simulink model "fw_sim"  (R2020a)
settings: Solver=ode4  StartTime=0.0  StopTime=45  FixedStep=0.01  RelTol=1e-3  EnableMultiTasking=on
undefined symbols (not defined in the file): ic_ned, ic_pqr, ic_rpy, ic_u, ic_uvw, wind
settings Model: Creator=fmina  LastModifiedBy=Chenhao
settings DataIOCC: SaveFormat=StructureWithTime  ReturnWorkspaceOutputs=off
settings OptimizationCC: LifeSpan=inf
settings DebuggingCC: SFUnexpectedBacktrackingDiag=warning  SFNoUnconditionalDefaultTransitionDiag=warning  SFExecutionAtInitializationDiag=none  ArithmeticOperatorsInVariantConditions=warning
settings HardwareCC: ProdBitPerSizeT=32  ProdBitPerPtrDiffT=32  ProdWordSize=32  ProdHWDeviceType=Specified
settings SFSimCC: SimUseLocalCustomCode=off  CustomCodeUndefinedFunction=UseInterfaceOnly
settings RTWCC: RTWUseLocalCustomCode=off
settings CodeAppCC: StateflowObjectComments=on
settings GRTTargetCC: TargetLangStandard=C89/C90 (ANSI)
settings ConfigComp: CovMetricSettings=dw  CovHtmlReporting=on  CovSaveCumulativeToWorkspaceVar=on  CovSaveSingleToWorkspaceVar=on  CovExternalEMLEnable=off

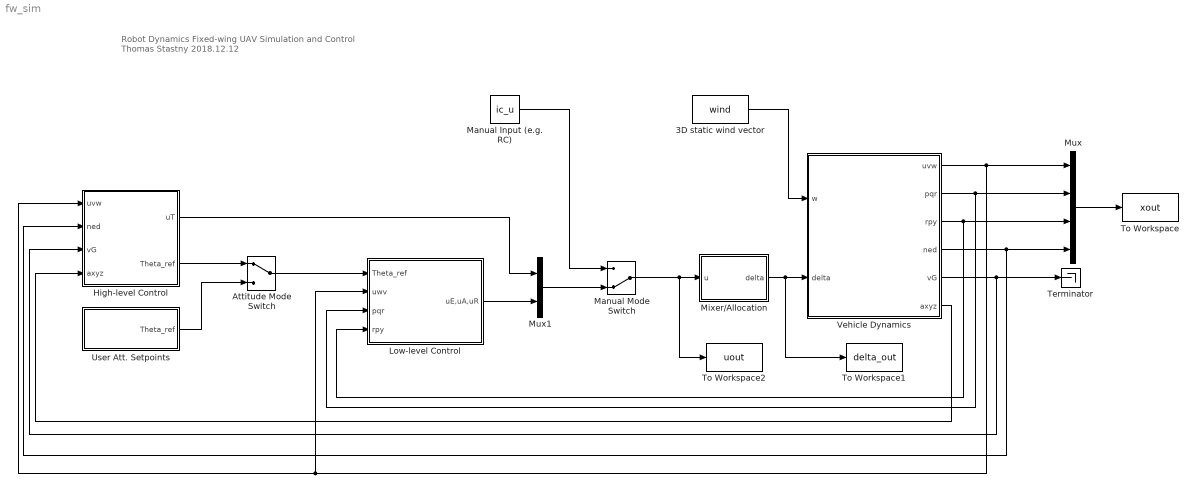
== system fw_sim ==
  note: Robot Dynamics
      | Fixed-wing UAV Simulation and Control
      |
      | Thomas Stastny
      | 2018.12.12
  3D static wind vector : Constant  Value=wind
  Attitude Mode Switch : ManualSwitch
  High-level Control : Subsystem
  Low-level Control : Subsystem
  Manual Input (e.g. RC) : Constant  Value=ic_u
  Manual Mode Switch : ManualSwitch  CurrentSetting=0
  Mixer/Allocation : MATLAB Function  TreatAsAtomicUnit=on
  Mux : Mux
  Mux1 : Mux  Inputs=2
  Terminator : Terminator
  To Workspace : ToWorkspace  VariableName=xout  SaveFormat=Structure With Time  SampleTime=-1
  To Workspace1 : ToWorkspace  VariableName=delta_out  SaveFormat=Structure With Time  SampleTime=-1
  To Workspace2 : ToWorkspace  VariableName=uout  SaveFormat=Structure With Time  SampleTime=-1
  User Att. Setpoints : Subsystem
  Vehicle Dynamics : Subsystem
  wires:
  3D static wind vector/1 -> Vehicle Dynamics/1(w)
  Mixer/Allocation/1(delta) -> To Workspace1/1, Vehicle Dynamics/2(delta)
  Mux/1 -> To Workspace/1
  Vehicle Dynamics/4(ned) -> High-level Control/2(ned), Mux/4
  Vehicle Dynamics/3(rpy) -> Low-level Control/4(rpy), Mux/3
  Vehicle Dynamics/1(uvw) -> Mux/1, Low-level Control/2(uwv), High-level Control/1(uvw)
  Vehicle Dynamics/2(pqr) -> Low-level Control/3(pqr), Mux/2
  Vehicle Dynamics/5(vG) -> High-level Control/3(vG), Terminator/1
  High-level Control/1(uT) -> Mux1/1
  Low-level Control/1(uE,uA,uR) -> Mux1/2
  Manual Mode Switch/1 -> To Workspace2/1, Mixer/Allocation/1(u)
  Manual Input (e.g. RC)/1 -> Manual Mode Switch/1
  Mux1/1 -> Manual Mode Switch/2
  Vehicle Dynamics/6(axyz) -> High-level Control/4(axyz)
  Attitude Mode Switch/1 -> Low-level Control/1(Theta_ref)
  High-level Control/2(Theta_ref) -> Attitude Mode Switch/1
  User Att. Setpoints/1(Theta_ref) -> Attitude Mode Switch/2

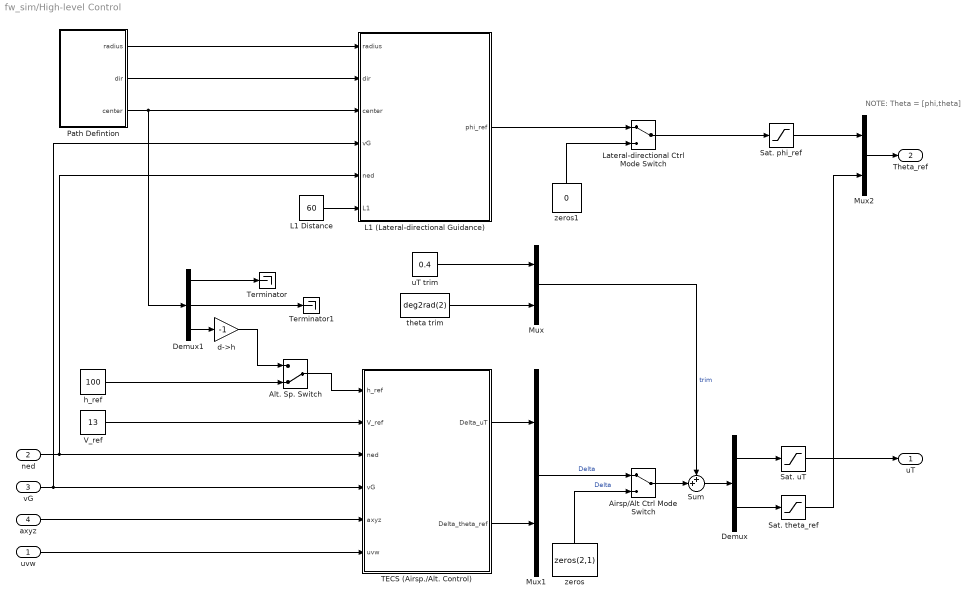
== system fw_sim/High-level Control ==
  note: NOTE: Theta = [phi,theta]
  uvw : Inport
  ned : Inport  Port=2
  vG : Inport  Port=3
  axyz : Inport  Port=4
  Airsp/Alt Ctrl Mode Switch : ManualSwitch
  Alt. Sp. Switch : ManualSwitch  CurrentSetting=0
  Demux : Demux  Outputs=2
  Demux1 : Demux  Outputs=3
  L1 (Lateral-directional Guidance) : MATLAB Function  TreatAsAtomicUnit=on
  L1 Distance : Constant  Value=60
  Lateral-directional Ctrl Mode Switch : ManualSwitch
  Mux : Mux  Inputs=2
  Mux1 : Mux  Inputs=2
  Mux2 : Mux  Inputs=2
  Path Defintion : Subsystem
  Sat. phi_ref : Saturate  UpperLimit=deg2rad(30)  LowerLimit=deg2rad(-30)
  Sat. theta_ref : Saturate  UpperLimit=deg2rad(15)  LowerLimit=deg2rad(-15)
  Sat. uT : Saturate  UpperLimit=1  LowerLimit=0
  Sum : Sum  Inputs=++|
  TECS (Airsp./Alt. Control) : Subsystem
  Terminator : Terminator
  Terminator1 : Terminator
  V_ref : Constant  Value=13
  d->h : Gain  Gain=-1
  h_ref : Constant  Value=100
  theta trim : Constant  Value=deg2rad(2)
  uT trim : Constant  Value=0.4
  zeros : Constant  Value=zeros(2,1)
  zeros1 : Constant  Value=0
  uT : Outport
  Theta_ref : Outport  Port=2
  wires:
  axyz/1 -> TECS (Airsp./Alt. Control)/5(axyz)
  vG/1 -> L1 (Lateral-directional Guidance)/4(vG), TECS (Airsp./Alt. Control)/4(vG)
  ned/1 -> L1 (Lateral-directional Guidance)/5(ned), TECS (Airsp./Alt. Control)/3(ned)
  uvw/1 -> TECS (Airsp./Alt. Control)/6(uvw)
  V_ref/1 -> TECS (Airsp./Alt. Control)/2(V_ref)
  uT trim/1 -> Mux/1
  theta trim/1 -> Mux/2
  TECS (Airsp./Alt. Control)/2(Delta_theta_ref) -> Mux1/2
  TECS (Airsp./Alt. Control)/1(Delta_uT) -> Mux1/1
  zeros/1 -> Airsp/Alt Ctrl Mode Switch/2  "Delta"
  Mux1/1 -> Airsp/Alt Ctrl Mode Switch/1  "Delta"
  Mux/1 -> Sum/1  "trim"
  Airsp/Alt Ctrl Mode Switch/1 -> Sum/2
  Sum/1 -> Demux/1
  Demux/1 -> Sat. uT/1
  Demux/2 -> Sat. theta_ref/1
  Sat. theta_ref/1 -> Mux2/2
  Sat. uT/1 -> uT/1
  Sat. phi_ref/1 -> Mux2/1
  Mux2/1 -> Theta_ref/1
  Path Defintion/3(center) -> Demux1/1, L1 (Lateral-directional Guidance)/3(center)
  Alt. Sp. Switch/1 -> TECS (Airsp./Alt. Control)/1(h_ref)
  h_ref/1 -> Alt. Sp. Switch/2
  Demux1/1 -> Terminator/1
  Demux1/2 -> Terminator1/1
  Demux1/3 -> d->h/1
  d->h/1 -> Alt. Sp. Switch/1
  Path Defintion/1(radius) -> L1 (Lateral-directional Guidance)/1(radius)
  Path Defintion/2(dir) -> L1 (Lateral-directional Guidance)/2(dir)
  L1 Distance/1 -> L1 (Lateral-directional Guidance)/6(L1)
  Lateral-directional Ctrl Mode Switch/1 -> Sat. phi_ref/1
  L1 (Lateral-directional Guidance)/1(phi_ref) -> Lateral-directional Ctrl Mode Switch/1
  zeros1/1 -> Lateral-directional Ctrl Mode Switch/2

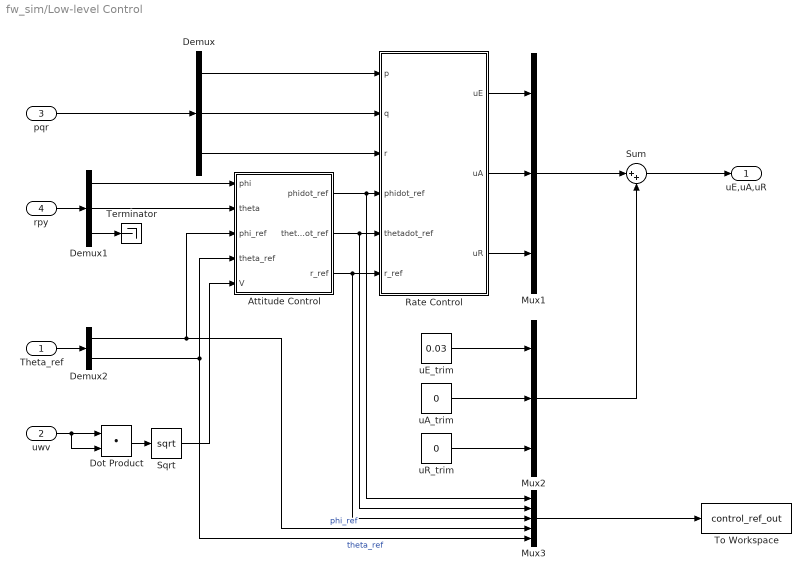
== system fw_sim/Low-level Control ==
  Theta_ref : Inport
  uwv : Inport  Port=2
  pqr : Inport  Port=3
  rpy : Inport  Port=4
  Attitude Control : Subsystem
  Demux : Demux  Outputs=3
  Demux1 : Demux  Outputs=3
  Demux2 : Demux  Outputs=2
  Dot Product : DotProduct  InputSameDT=on  OutDataTypeStr=Inherit: Inherit via internal rule
  Mux1 : Mux  Inputs=3
  Mux2 : Mux  Inputs=3
  Mux3 : Mux  Inputs=5
  Rate Control : Subsystem
  Sqrt : Sqrt  SaturateOnIntegerOverflow=on
  Sum : Sum  Inputs=|++
  Terminator : Terminator
  To Workspace : ToWorkspace  VariableName=control_ref_out  SaveFormat=Structure With Time  SampleTime=-1
  uA_trim : Constant  Value=0
  uE_trim : Constant  Value=0.03
  uR_trim : Constant  Value=0
  uE,uA,uR : Outport
  wires:
  Attitude Control/1(phidot_ref) -> Mux3/1, Rate Control/4(phidot_ref)
  Rate Control/2("uA ") -> Mux1/2
  Attitude Control/3(r_ref) -> Mux3/3, Rate Control/6(r_ref)
  Demux2/2 -> Mux3/5, Attitude Control/4(theta_ref)  "theta_ref"
  Attitude Control/2(thetadot_ref) -> Mux3/2, Rate Control/5(thetadot_ref)
  Rate Control/3(uR) -> Mux1/3
  Rate Control/1(uE) -> Mux1/1
  Demux/2 -> Rate Control/2(q)
  Demux/3 -> Rate Control/3(r)
  Demux/1 -> Rate Control/1(p)
  pqr/1 -> Demux/1
  rpy/1 -> Demux1/1
  Demux1/1 -> Attitude Control/1(phi)
  Demux1/2 -> Attitude Control/2(theta)
  Demux1/3 -> Terminator/1
  Dot Product/1 -> Sqrt/1
  uwv/1 -> Dot Product/2, Dot Product/1
  Sqrt/1 -> Attitude Control/5(V)
  uE_trim/1 -> Mux2/1
  uA_trim/1 -> Mux2/2
  uR_trim/1 -> Mux2/3
  Mux2/1 -> Sum/2
  Mux1/1 -> Sum/1
  Sum/1 -> uE,uA,uR/1
  Mux3/1 -> To Workspace/1
  Demux2/1 -> Mux3/4, Attitude Control/3(phi_ref)  "phi_ref"
  Theta_ref/1 -> Demux2/1

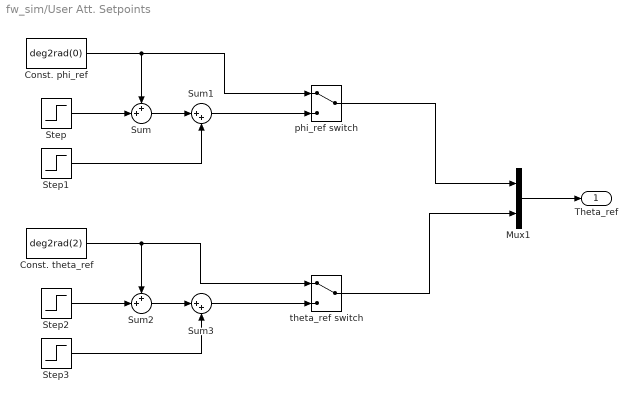
== system fw_sim/User Att. Setpoints ==
  Const. phi_ref : Constant  Value=deg2rad(0)
  Const. theta_ref : Constant  Value=deg2rad(2)
  Mux1 : Mux  Inputs=2
  Step : Step  Time=5  After=deg2rad(20)  SampleTime=0
  Step1 : Step  Time=7  After=deg2rad(-20)  SampleTime=0
  Step2 : Step  Time=5  After=deg2rad(7)  SampleTime=0
  Step3 : Step  Time=7  After=deg2rad(-7)  SampleTime=0
  Sum : Sum  Inputs=++|
  Sum1 : Sum  Inputs=|++
  Sum2 : Sum  Inputs=++|
  Sum3 : Sum  Inputs=|++
  phi_ref switch : ManualSwitch
  theta_ref switch : ManualSwitch
  Theta_ref : Outport
  wires:
  Step/1 -> Sum/2
  Sum/1 -> Sum1/1
  Step1/1 -> Sum1/2
  Const. phi_ref/1 -> phi_ref switch/1, Sum/1
  Mux1/1 -> Theta_ref/1
  Sum1/1 -> phi_ref switch/2
  Step2/1 -> Sum2/2
  Sum2/1 -> Sum3/1
  Step3/1 -> Sum3/2
  Const. theta_ref/1 -> Sum2/1, theta_ref switch/1
  Sum3/1 -> theta_ref switch/2
  phi_ref switch/1 -> Mux1/1
  theta_ref switch/1 -> Mux1/2

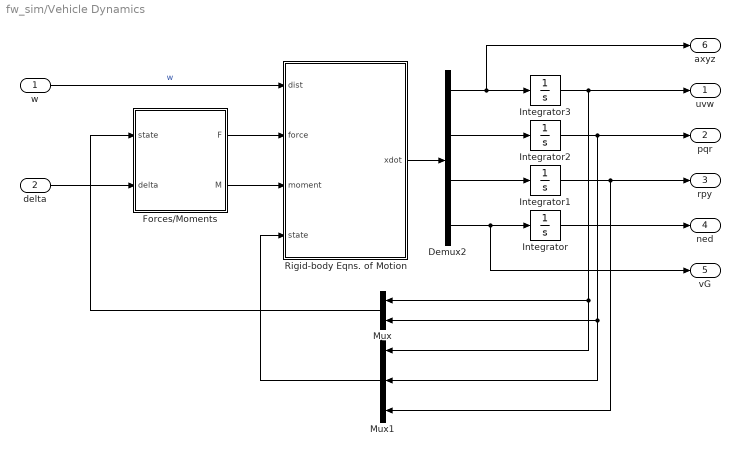
== system fw_sim/Vehicle Dynamics ==
  w : Inport
  delta : Inport  Port=2
  Demux2 : Demux
  Forces/Moments : MATLAB Function  TreatAsAtomicUnit=on
  Integrator : Integrator  InitialCondition=ic_ned
  Integrator1 : Integrator  InitialCondition=ic_rpy
  Integrator2 : Integrator  InitialCondition=ic_pqr
  Integrator3 : Integrator  InitialCondition=ic_uvw
  Mux : Mux  Inputs=2
  Mux1 : Mux  Inputs=3
  Rigid-body Eqns. of Motion : MATLAB Function  TreatAsAtomicUnit=on
  uvw : Outport
  pqr : Outport  Port=2
  rpy : Outport  Port=3
  ned : Outport  Port=4
  vG : Outport  Port=5
  axyz : Outport  Port=6
  wires:
  w/1 -> Rigid-body Eqns. of Motion/1(dist)  "w"
  Mux/1 -> Forces/Moments/1(state)
  delta/1 -> Forces/Moments/2(delta)
  Forces/Moments/1(F) -> Rigid-body Eqns. of Motion/2(force)
  Forces/Moments/2(M) -> Rigid-body Eqns. of Motion/3(moment)
  Rigid-body Eqns. of Motion/1(xdot) -> Demux2/1
  Demux2/1 -> axyz/1, Integrator3/1
  Integrator/1 -> ned/1
  Demux2/4 -> vG/1, Integrator/1
  Demux2/3 -> Integrator1/1
  Demux2/2 -> Integrator2/1
  Integrator3/1 -> Mux1/1, Mux/1, uvw/1
  Integrator2/1 -> Mux1/2, Mux/2, pqr/1
  Integrator1/1 -> Mux1/3, rpy/1
  Mux1/1 -> Rigid-body Eqns. of Motion/4(state)

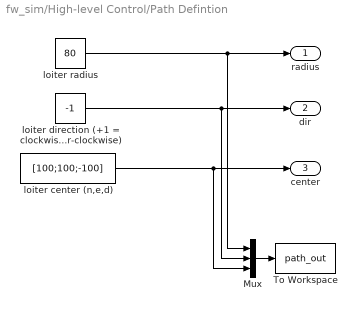
== system fw_sim/High-level Control/Path Defintion ==
  Mux : Mux  Inputs=3
  To Workspace : ToWorkspace  VariableName=path_out  SaveFormat=Structure With Time  SampleTime=-1
  loiter center (n,e,d) : Constant  Value=[100;100;-100]
  "loiter direction (+1 = clockwise, -1 = counter-clockwise)" : Constant  Value=-1
  loiter radius : Constant  Value=80
  radius : Outport
  dir : Outport  Port=2
  center : Outport  Port=3
  wires:
  loiter radius/1 -> Mux/1, radius/1
  loiter center (n,e,d)/1 -> Mux/3, center/1
  "loiter direction (+1 = clockwise, -1 = counter-clockwise)"/1 -> Mux/2, dir/1
  Mux/1 -> To Workspace/1

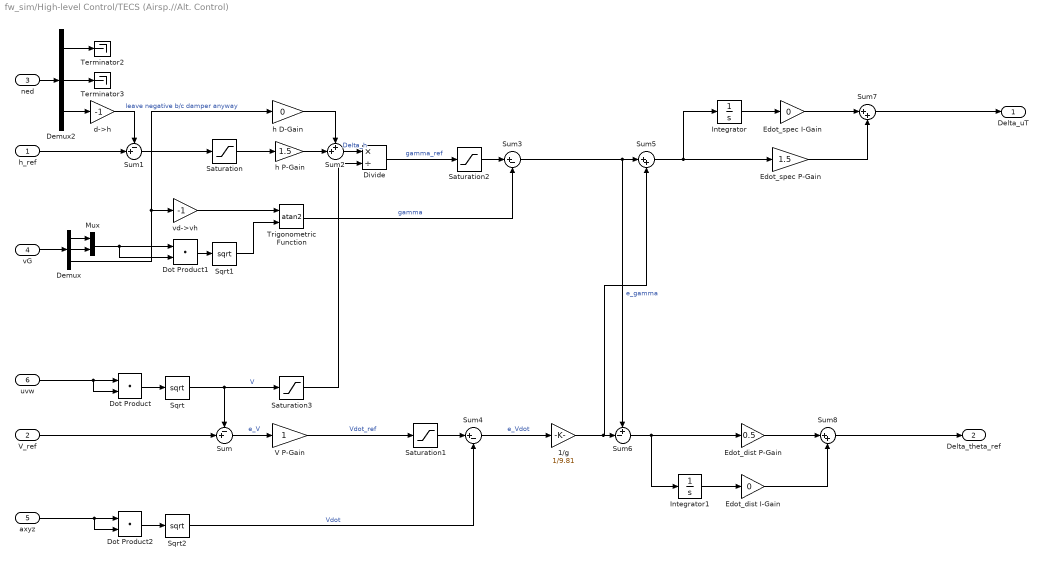
== system fw_sim/High-level Control/TECS (Airsp.//Alt. Control) ==
  h_ref : Inport
  V_ref : Inport  Port=2
  ned : Inport  Port=3
  vG : Inport  Port=4
  axyz : Inport  Port=5
  uvw : Inport  Port=6
  1/g : Gain  Gain=1/9.81
  Demux : Demux  Outputs=3
  Demux2 : Demux  Outputs=3
  Divide : Product  Inputs=*/
  Dot Product : DotProduct  InputSameDT=on  OutDataTypeStr=Inherit: Inherit via internal rule
  Dot Product1 : DotProduct  InputSameDT=on  OutDataTypeStr=Inherit: Inherit via internal rule
  Dot Product2 : DotProduct  InputSameDT=on  OutDataTypeStr=Inherit: Inherit via internal rule
  Edot_dist I-Gain : Gain  Gain=0
  Edot_dist P-Gain : Gain  Gain=0.5
  Edot_spec I-Gain : Gain  Gain=0
  Edot_spec P-Gain : Gain  Gain=1.5
  Integrator : Integrator
  Integrator1 : Integrator
  Mux : Mux  Inputs=2
  Saturation : Saturate  UpperLimit=10  LowerLimit=-10
  Saturation1 : Saturate  UpperLimit=10  LowerLimit=-10
  Saturation2 : Saturate  UpperLimit=deg2rad(15)  LowerLimit=deg2rad(-15)
  Saturation3 : Saturate  UpperLimit=20  LowerLimit=5
  Sqrt : Sqrt  SaturateOnIntegerOverflow=on
  Sqrt1 : Sqrt  SaturateOnIntegerOverflow=on
  Sqrt2 : Sqrt  SaturateOnIntegerOverflow=on
  Sum : Sum  Inputs=-+|
  Sum1 : Sum  Inputs=-+|
  Sum2 : Sum  Inputs=++|
  Sum3 : Sum  Inputs=|+-
  Sum4 : Sum  Inputs=|+-
  Sum5 : Sum  Inputs=|++
  Sum6 : Sum  Inputs=+-|
  Sum7 : Sum  Inputs=|++
  Sum8 : Sum  Inputs=|++
  Terminator2 : Terminator
  Terminator3 : Terminator
  Trigonometric Function : Trigonometry  Operator=atan2
  V P-Gain : Gain
  d->h : Gain  Gain=-1
  h D-Gain : Gain  Gain=0
  h P-Gain : Gain  Gain=1.5
  vd->vh : Gain  Gain=-1
  Delta_uT : Outport
  Delta_theta_ref : Outport  Port=2
  wires:
  Dot Product/1 -> Sqrt/1
  vG/1 -> Demux/1
  Dot Product1/1 -> Sqrt1/1
  Sqrt1/1 -> Trigonometric Function/2
  Demux/3 -> vd->vh/1, h D-Gain/1  "leave negative b/c damper anyway"
  Sqrt/1 -> Saturation3/1, Sum/1  "V"
  V_ref/1 -> Sum/2
  Sum/1 -> V P-Gain/1  "e_V"
  h_ref/1 -> Sum1/2
  Sum1/1 -> Saturation/1
  Saturation/1 -> h P-Gain/1
  h P-Gain/1 -> Sum2/2
  Sum2/1 -> Divide/1  "Delta_h"
  Trigonometric Function/1 -> Sum3/2  "gamma"
  axyz/1 -> Dot Product2/2, Dot Product2/1
  V P-Gain/1 -> Saturation1/1  "Vdot_ref"
  Sum4/1 -> 1/g/1  "e_Vdot"
  Sum3/1 -> Sum5/1, Sum6/1  "e_gamma"
  1/g/1 -> Sum6/2, Sum5/2
  Sum5/1 -> Integrator/1, Edot_spec P-Gain/1
  Sum6/1 -> Integrator1/1, Edot_dist P-Gain/1
  Integrator/1 -> Edot_spec I-Gain/1
  Integrator1/1 -> Edot_dist I-Gain/1
  Edot_spec I-Gain/1 -> Sum7/1
  Edot_spec P-Gain/1 -> Sum7/2
  Edot_dist P-Gain/1 -> Sum8/1
  Edot_dist I-Gain/1 -> Sum8/2
  uvw/1 -> Dot Product/2, Dot Product/1
  ned/1 -> Demux2/1
  Demux2/3 -> d->h/1
  d->h/1 -> Sum1/1
  Demux2/2 -> Terminator3/1
  Demux2/1 -> Terminator2/1
  vd->vh/1 -> Trigonometric Function/1
  Saturation2/1 -> Sum3/1
  h D-Gain/1 -> Sum2/1
  Sum7/1 -> Delta_uT/1
  Sum8/1 -> Delta_theta_ref/1
  Sqrt2/1 -> Sum4/2  "Vdot"
  Dot Product2/1 -> Sqrt2/1
  Demux/1 -> Mux/1
  Demux/2 -> Mux/2
  Mux/1 -> Dot Product1/1, Dot Product1/2
  Saturation1/1 -> Sum4/1
  Divide/1 -> Saturation2/1  "gamma_ref"
  Saturation3/1 -> Divide/2

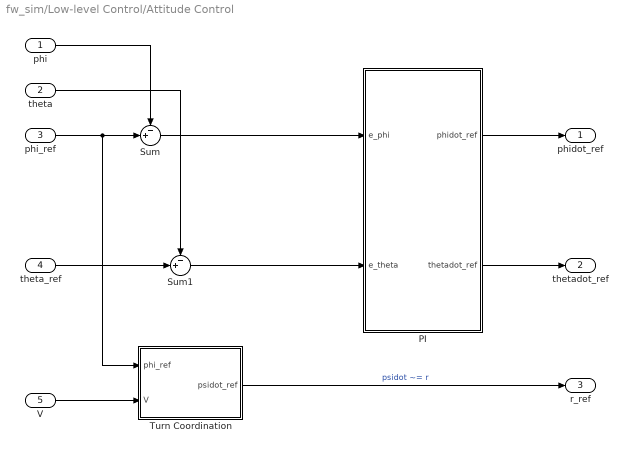
== system fw_sim/Low-level Control/Attitude Control ==
  phi : Inport
  theta : Inport  Port=2
  phi_ref : Inport  Port=3
  theta_ref : Inport  Port=4
  V : Inport  Port=5
  PI : Subsystem
  Sum : Sum  Inputs=-+|
  Sum1 : Sum  Inputs=-+|
  Turn Coordination : Subsystem
  phidot_ref : Outport
  thetadot_ref : Outport  Port=2
  r_ref : Outport  Port=3
  wires:
  PI/1(phidot_ref) -> phidot_ref/1
  PI/2(thetadot_ref) -> thetadot_ref/1
  Turn Coordination/1(psidot_ref) -> r_ref/1  "psidot ~= r"
  phi/1 -> Sum/1
  theta/1 -> Sum1/1
  phi_ref/1 -> Turn Coordination/1(phi_ref), Sum/2
  Sum/1 -> PI/1(e_phi)
  theta_ref/1 -> Sum1/2
  V/1 -> Turn Coordination/2(V)
  Sum1/1 -> PI/2(e_theta)

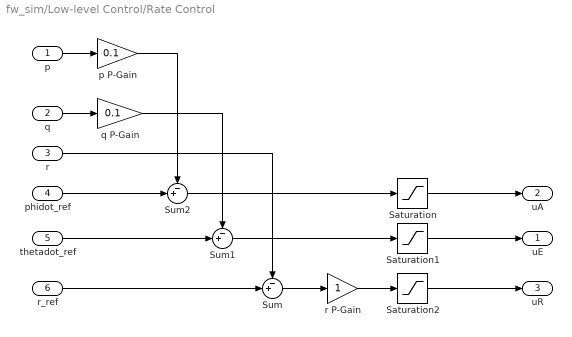
== system fw_sim/Low-level Control/Rate Control ==
  p : Inport
  q : Inport  Port=2
  r : Inport  Port=3
  phidot_ref : Inport  Port=4
  thetadot_ref : Inport  Port=5
  r_ref : Inport  Port=6
  Saturation : Saturate  UpperLimit=1  LowerLimit=-1
  Saturation1 : Saturate  UpperLimit=1  LowerLimit=-1
  Saturation2 : Saturate  UpperLimit=1  LowerLimit=-1
  Sum : Sum  Inputs=-+|
  Sum1 : Sum  Inputs=-+|
  Sum2 : Sum  Inputs=-+|
  p P-Gain : Gain  Gain=0.1
  q P-Gain : Gain  Gain=0.1
  r P-Gain : Gain
  uE : Outport
  "uA " : Outport  Port=2
  uR : Outport  Port=3
  wires:
  p/1 -> p P-Gain/1
  q/1 -> q P-Gain/1
  r/1 -> Sum/1
  phidot_ref/1 -> Sum2/2
  thetadot_ref/1 -> Sum1/2
  r_ref/1 -> Sum/2
  Sum/1 -> r P-Gain/1
  Sum2/1 -> Saturation/1
  Saturation/1 -> "uA "/1
  Sum1/1 -> Saturation1/1
  Saturation1/1 -> uE/1
  Saturation2/1 -> uR/1
  r P-Gain/1 -> Saturation2/1
  p P-Gain/1 -> Sum2/1
  q P-Gain/1 -> Sum1/1

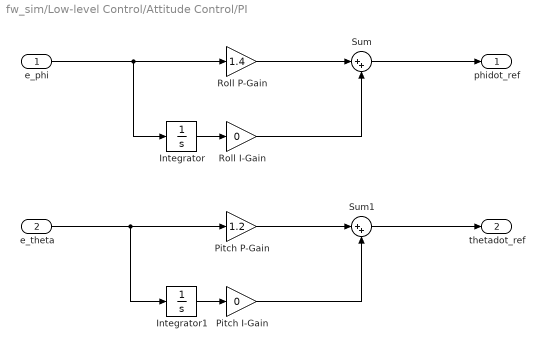
== system fw_sim/Low-level Control/Attitude Control/PI ==
  e_phi : Inport
  e_theta : Inport  Port=2
  Integrator : Integrator
  Integrator1 : Integrator
  Pitch I-Gain : Gain  Gain=0
  Pitch P-Gain : Gain  Gain=1.2
  Roll I-Gain : Gain  Gain=0
  Roll P-Gain : Gain  Gain=1.4
  Sum : Sum  Inputs=|++
  Sum1 : Sum  Inputs=|++
  phidot_ref : Outport
  thetadot_ref : Outport  Port=2
  wires:
  e_phi/1 -> Integrator/1, Roll P-Gain/1
  Integrator/1 -> Roll I-Gain/1
  e_theta/1 -> Integrator1/1, Pitch P-Gain/1
  Integrator1/1 -> Pitch I-Gain/1
  Roll P-Gain/1 -> Sum/1
  Roll I-Gain/1 -> Sum/2
  Sum/1 -> phidot_ref/1
  Pitch P-Gain/1 -> Sum1/1
  Sum1/1 -> thetadot_ref/1
  Pitch I-Gain/1 -> Sum1/2

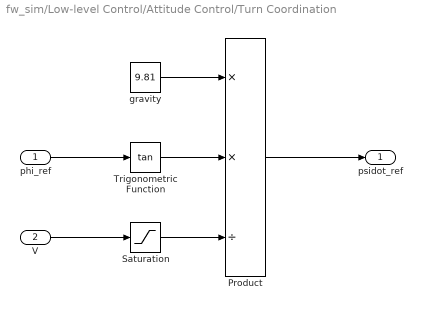
== system fw_sim/Low-level Control/Attitude Control/Turn Coordination ==
  phi_ref : Inport
  V : Inport  Port=2
  Product : Product  Inputs=**/
  Saturation : Saturate  UpperLimit=20  LowerLimit=5
  Trigonometric Function : Trigonometry  Operator=tan
  gravity : Constant  Value=9.81
  psidot_ref : Outport
  wires:
  gravity/1 -> Product/1
  V/1 -> Saturation/1
  phi_ref/1 -> Trigonometric Function/1
  Trigonometric Function/1 -> Product/2
  Product/1 -> psidot_ref/1
  Saturation/1 -> Product/3

== matlab function fw_sim/Mixer//Allocation ==
  data: u input; delta output
function delta = fcn(u)

% LOAD PARAMETERS
params = parameters();

% INPUT TO DEFLECTION
delta = zeros(5,1);
delta(1) = u(1);                    % throttle
delta(2) = u(2) * params.deltamax;  % elevator
delta(3) = u(3) * params.deltamax;  % aileron right
delta(4) = -u(3) * params.deltamax; % aileron left
delta(5) = u(4) * params.deltamax;  % rudder

== matlab function fw_sim/Vehicle Dynamics/Forces//Moments ==
  data: state input; F output; delta input; M output
function [F,M] = fcn(state,delta)

% LOAD PARAMETERS
params = parameters();

% STATES
u = state(1);       % x-body velocity
v = state(2);       % y-body velocity
w = state(3);       % z-body velocity
p = state(4);       % roll rate
q = state(5);       % pitch rate
r = state(6);       % yaw rate

% intermediate states (wind-frame)
VA = sqrt(u^2+v^2+w^2);
alpha = atan2(w,u); % angle of attack
beta = asin(v/VA);

% DEFLECTIONS
deltaT = delta(1);
deltaE = delta(2);
deltaA_R = delta(3);
deltaA_L = delta(4);
deltaR = delta(5);

% stability-to-body transform
ca = cos(alpha);
sa = sin(alpha);
H_S2B = [ca, 0, -sa; 0, 1, 0; sa, 0, ca];

% non-dimensionalized rates
p_hat = p*params.b /(2*14);
q_hat = q*params.c /(2*14);
r_hat = r*params.b /(2*14);
q_bar_S = 0.5*params.rho*VA^2*params.S;

% aerodynamic force coefficients (stability-axis)
% component build-up
cD = params.cD0 + params.cDa*alpha + params.cDa2*alpha^2;
cY_s = 0*params.cYb*beta;
cL  = params.cL0 + params.cLa*alpha + params.cLa2*alpha^2 + ...
    params.cLa3*alpha^3 + params.cLq*q_hat + params.cLde*deltaE;

% aerodynamic moment coefficients (stability-axis)
% component build-up
cl_s = params.clb*beta + params.clp*p_hat + params.clr*r_hat + params.clda*deltaA_R - params.clda*deltaA_L;
cm_s = params.cm0 + params.cma*alpha + params.cmq*q_hat + params.cmde*deltaE;
cn_s = params.cnb*beta + params.cnp*p_hat + params.cnr*r_hat + params.cndr*deltaR;

% AERODYNAMIC FORCES (body-frame)
FA = q_bar_S * H_S2B*[-cD; cY_s; -cL];
     
% THRUST FORCE (body-frame)
FT = (params.cT0 + params.cT1*deltaT + params.cT2*deltaT^2) * ...
    [cos(params.epsilon); 0; sin(params.epsilon)];

% AERODYNAMIC MOMENTS (body-frame)
MA = q_bar_S * diag([params.b, params.c, params.b]) * [cl_s; cm_s; cn_s];

% THRUST MOMENTS (body-frame)
MT = zeros(3,1);

F = FA + FT;
M = MA + MT;

== matlab function fw_sim/Vehicle Dynamics/Rigid-body Eqns. of Motion ==
  data: dist input; force input; moment input; state input; xdot output
function xdot = fcn(dist,force,moment,state)

params = parameters();

% DISTURBANCE
wn = dist(1);       % northing wind
we = dist(2);       % easting wind
wd = dist(3);       % down wind

% FORCES / MOMENTS
X = force(1);       % summed forces on x-body axis
Y = force(2);       % summed forces on y-body axis
Z = force(3);       % summed forces on z-body axis
Lm = moment(1);     % summed moments about x-body axis
Mm = moment(2);     % summed moments about y-body axis
Nm = moment(3);     % summed moments about z-body axis

% STATES
u = state(1);       % x-body velocity
v = state(2);       % y-body velocity
w = state(3);       % z-body velocity
p = state(4);       % roll rate
q = state(5);       % pitch rate
r = state(6);       % yaw rate
phi = state(7);     % roll angle
theta = state(8);   % pitch angle
psi = state(9);     % yaw angle

% TRANSLATIONAL DYNAMICS

% u,v,w
udot = r*v - q*w - params.g*sin(theta) + X/params.mass;
vdot = p*w - r*u + params.g*sin(phi)*cos(theta) + Y/params.mass;
wdot = q*u - p*v + params.g*cos(phi)*cos(theta) + Z/params.mass;

% n,e,d
ndot = u*cos(theta)*cos(psi)+v*(sin(phi)*sin(theta)*cos(psi)-...
    cos(phi)*sin(psi))+w*(sin(phi)*sin(psi)+cos(phi)*sin(theta)*cos(psi)) + wn;
edot = u*cos(theta)*sin(psi)+v*(cos(phi)*cos(psi)+sin(phi)*sin(theta)*sin(psi))+...
    w*(cos(phi)*sin(theta)*sin(psi)-sin(phi)*cos(psi)) + we;
ddot = -u*sin(theta)+v*sin(phi)*cos(theta)+w*cos(phi)*cos(theta) + wd;

% ROTATIONAL DYNAMICS

% p,q,r
pdot = (Lm+(params.Iyy-params.Izz)*r*q)/params.Ixx;
qdot = (Mm+(params.Izz-params.Ixx)*p*r)/params.Iyy;
rdot = (Nm+(params.Ixx-params.Iyy)*p*q)/params.Izz;

% phi,theta,psi
phidot = p + (q*sin(phi) + r*cos(phi))*tan(theta);
thetadot = q*cos(phi) - r*sin(phi);
psidot = (q*sin(phi) + r*cos(phi))/cos(theta);

% STATE DIFFERENTIALS
xdot = [udot;vdot;wdot;pdot;qdot;rdot;phidot;thetadot;psidot;ndot;edot;ddot];

== matlab function fw_sim/High-level Control/L1 (Lateral-directional Guidance) ==
  data: radius input size=1; phi_ref output size=1; dir input size=1; center input size=3; vG input size=3; ned input size=3; L1 input size=1
function phi_ref = fcn(radius,dir,center,vG,ned,L1)

% calculate lateral-directional ground speed
ground_speed = norm(vG(1:2,1));

% vector from position to center of loiter
v_ned_to_center = center(1:2,1)-ned(1:2,1);
ned_to_center_bearing = atan2(v_ned_to_center(2),v_ned_to_center(1));

% calculate the distance from the aircraft to the circle
dist2circ = norm(v_ned_to_center)-radius;
abs_dist2circ = abs(dist2circ);

% check that L1 vector does not exceed reasonable bounds
if L1 >= (2*radius + dist2circ)
    L1 = 2*radius + dist2circ;
elseif L1 < abs_dist2circ
    L1 = abs_dist2circ;
end

% calculate L1 bearing (law of cosines)
cos_gam = (L1^2 + (dist2circ + radius)^2 - radius^2) ...
    / 2 / L1 / (dist2circ + radius);
if cos_gam > 1, cos_gam = 1; end
if cos_gam < -1, cos_gam = -1; end;
gam = acos(cos_gam);
L1_bearing = ned_to_center_bearing - dir * gam;
if (L1_bearing>pi), L1_bearing = L1_bearing - 2*pi; end;
if (L1_bearing<-pi), L1_bearing = L1_bearing + 2*pi; end;

% calculate error angle eta
ground_speed_bearing = atan2(vG(2,1), vG(1,1));
eta = L1_bearing - ground_speed_bearing;
if (eta>pi), eta = eta - 2*pi; end;
if (eta<-pi), eta = eta + 2*pi; end;

% limit eta to 90 degrees
if (eta>pi/2), eta = pi/2; end;
if (eta<-pi/2), eta = -pi/2; end;

% normal acceleration reference
aN_ref = 2*ground_speed^2*sin(eta)/L1;

% coordinated roll mapping
phi_ref = atan(aN_ref/9.81);
